simulink model "ziegler_PID_one"  (R2018a)
settings: Solver=VariableStepAuto  StartTime=0.0  StopTime=1000.0  RelTol=1e-3
libraries: simulink_extras x1
settings Model: Creator=benko  LastModifiedBy=benko

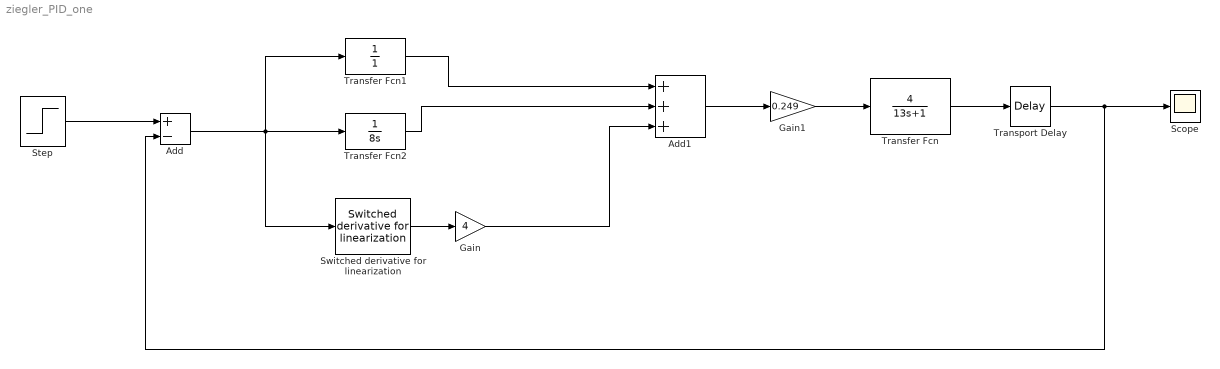
== system ziegler_PID_one ==
  Add : Sum  Inputs=+-
  Add1 : Sum  Inputs=+++
  Gain : Gain  Gain=4
  Gain1 : Gain  Gain=0.249
  Scope : Scope
  Step : Step  SampleTime=0
  Switched derivative for linearization : simulink_extras/Linearization/Switched derivative for linearization  switchVal=0  derivConst=100
      settings: SourceProductName=Simulink  SourceProductBaseCode=SL
  Transfer Fcn : TransferFcn  Numerator=4  Denominator=[13 1]
  Transfer Fcn1 : TransferFcn  Numerator=1  Denominator=1
  Transfer Fcn2 : TransferFcn  Denominator=[8 0]
  Transport Delay : TransportDelay  DelayTime=4
  wires:
  Transfer Fcn/1 -> Transport Delay/1
  Transport Delay/1 -> Add/2, Scope/1
  Switched derivative for linearization/1 -> Gain/1
  Step/1 -> Add/1
  Add/1 -> Transfer Fcn1/1, Transfer Fcn2/1, Switched derivative for linearization/1
  Transfer Fcn1/1 -> Add1/1
  Transfer Fcn2/1 -> Add1/2
  Gain/1 -> Add1/3
  Gain1/1 -> Transfer Fcn/1
  Add1/1 -> Gain1/1
